simulink model "HevMmReferenceApplication"  (R2020a)
settings: Solver=ode23tb  StartTime=0  StopTime=2474  RelTol=1e-3  EnableMultiTasking=on
undefined symbols (not defined in the file): sigbuilder_block
libraries: autolibshared x2
(part 1 of 2)
settings Model: ModifiedByFormat=The MathWorks, Inc.  SimulationMode=accelerator  PauseTimes=23.46  Creator=The MathWorks, Inc.  LastModifiedBy=The MathWorks, Inc.
settings SolverCC: ZeroCrossAlgorithm=Adaptive  MinimalZcImpactIntegration=on
settings DataIOCC: DSMLogging=off  ReturnWorkspaceOutputs=off
settings DebuggingCC: UnderspecifiedInitializationDetection=Classic  MergeDetectMultiDrivingBlocksExec=none  MaskedZcDiagnostic=none  IgnoredZcDiagnostic=none  ModelReferenceExtraNoncontSigs=none  PregeneratedLibrarySubsystemCodeDiagnostic=none  ArithmeticOperatorsInVariantConditions=warning
settings ModelReferenceCC: UpdateModelReferenceTargets=IfOutOfDate  ModelReferenceMinAlgLoopOccurrences=on  PropagateSignalLabelsOutOfModel=off
settings SFSimCC: SimUseLocalCustomCode=off
settings RTWCC: RTWUseLocalCustomCode=off
settings CodeAppCC: StateflowObjectComments=on
settings GRTTargetCC: TargetLangStandard=C89/C90 (ANSI)
settings ConfigComp: CovMetricSettings=dsw  CovHtmlReporting=on  CovSaveCumulativeToWorkspaceVar=on  CovSaveSingleToWorkspaceVar=on  CovShowResultsExplorer=off  CovExternalEMLEnable=off

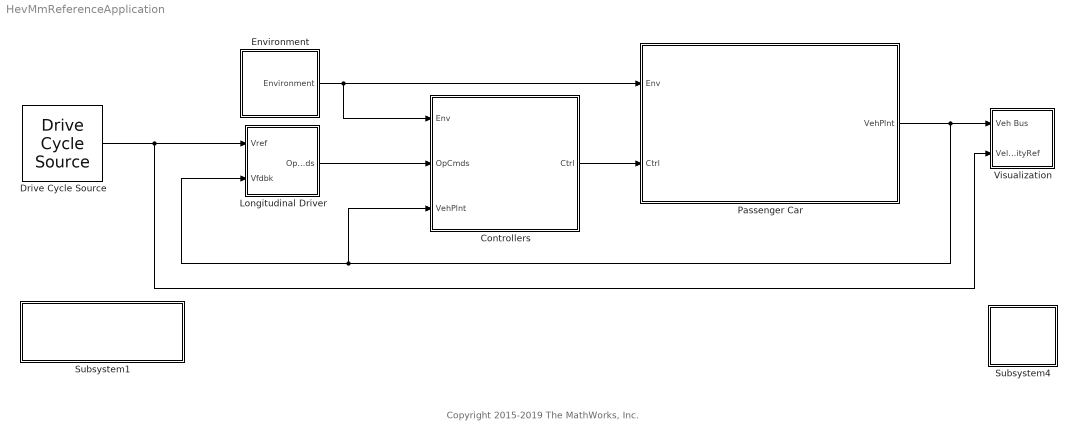
== system HevMmReferenceApplication ==
  note: Copyright 2015-2019 The MathWorks, Inc.
  Controllers : Subsystem
      mask Display: image('SystemControllers.png', 'center')
  Drive Cycle Source : autolibshared/Drive Cycle Source  cycleVar=FTP75  fileVar=L:\Bauto\matlab\test\toolbox\shared\autoblks\scenario\adac.txt  tfinal="2474  seconds"  cycleRepeat=off  outAccPort=off  outGearPort=off  gearList=No gear data  t_wot1=5  xdot_woto=0  xdot_wot1=30  t_wot2=20  xdot_wot2=0  t_wotend=30  srcUnit=m/s  outUnit=m/s  srcAccUnit=m/s/s  outAccUnit=m/s^2  dt=0  aMode=1  faultOption=off  velBnd=2  velBndUnit=mph  inUnit=m/s  timeBnd=1  failOption=off  stopSim=off  maxFaultCnt=10  maxFaultTime=2  maxTotFaultTime=15  traceOption=off  dtTrace=1  traceWindow=10  lastDCname=FTP75 Velocity  lastOutUnit=mph  lastDT=0  lastTB=1  lastSB=2  forceCalcBound=off
      settings: SourceProductBaseCode=PW,MT,VE,VP
  Environment : Subsystem
      mask Display: disp('Environment')
  Longitudinal Driver : Subsystem  Variant=on  VariantControlMode=Label  VariantControl=Variant1  LabelModeActiveChoice=0
      mask Display:
      | if strcmp('1',get_param(gcb,'ActiveVariant'))
      |     disp('Open Loop')
      | else
      |     image('LongitudinalDriver.png','center');
      | end
  Passenger Car : Subsystem
      mask Display: image('PassengerVehicle.png', 'center')
  Subsystem1 : Subsystem
      settings: OpenFcn=edit GenerateEnergyReport
      mask Display: disp('Analyze Power and Energy')
  Subsystem4 : Subsystem
      settings: OpenFcn=helpview([docroot,'/toolbox/autoblks/helptargets.map'], 'hybrid_refapp')
      mask Display: disp('Help')
  Visualization : Subsystem
      mask Display: disp('Visualization')
  wires:
  Longitudinal Driver/1(" OpCmds") -> Controllers/2(OpCmds)
  Drive Cycle Source/1 -> Longitudinal Driver/1("Vref "), Visualization/2(VelocityRef)
  Environment/1(Environment) -> Passenger Car/1(Env), Controllers/1(Env)
  Controllers/1(Ctrl) -> Passenger Car/2(Ctrl)
  Passenger Car/1(VehPlnt) -> Longitudinal Driver/2("Vfdbk "), Controllers/3(VehPlnt), Visualization/1(Veh Bus)

== system HevMmReferenceApplication/Controllers ==
  Env : Inport
  OpCmds : Inport  Port=2
  VehPlnt : Inport  Port=3
  Bus Creator : BusCreator  Inputs=2
  PCM Input : Subsystem
  PCM Output : Subsystem
  Powertrain Control Module (PCM) : Subsystem
  Ctrl : Outport  VectorParamsAs1DForOutWhenUnconnected=off
  wires:
  PCM Output/1(EngCtrl) -> [EngCtrl]
  Bus Creator/1 -> Ctrl/1
  [EngCtrl] -> Bus Creator/1
  [PtCtrl] -> Bus Creator/2
  Env/1 -> [Environment]
  [OpCmds] -> PCM Input/4(OpCmds)
  VehPlnt/1 -> [VehPlnt]
  OpCmds/1 -> [OpCmds]
  [PtCtrl] -> PCM Input/1(PtCtrl)
  [Environment] -> PCM Input/2(Env)
  [VehPlnt] -> PCM Input/3(VehPlnt)
  PCM Output/2(PtCtrl) -> [PtCtrl]
  PCM Input/1(TrqCmd) -> Powertrain Control Module (PCM)/1(TrqCmd)
  PCM Input/2(EngSpd) -> Powertrain Control Module (PCM)/2(EngSpd)
  PCM Input/3(Map) -> Powertrain Control Module (PCM)/3(Map)
  PCM Input/4(Mat) -> Powertrain Control Module (PCM)/4(Mat)
  PCM Input/5(ThrPosPct) -> Powertrain Control Module (PCM)/5(ThrPosPct)
  PCM Input/6(WgAreaPct) -> Powertrain Control Module (PCM)/6(WgAreaPct)
  PCM Input/7(IntkCamPhase) -> Powertrain Control Module (PCM)/7(IntkCamPhase)
  PCM Input/8(ExhCamPhase) -> Powertrain Control Module (PCM)/8(ExhCamPhase)
  PCM Input/9(TurboRackPos) -> Powertrain Control Module (PCM)/9(TurboRackPos)
  PCM Input/10(EgrVlvAreaPct) -> Powertrain Control Module (PCM)/10(EgrVlvAreaPct)
  PCM Input/11(VarCompRatioPos) -> Powertrain Control Module (PCM)/11(VarCompRatioPos)
  PCM Input/12(IntkVlvLift) -> Powertrain Control Module (PCM)/12(IntkVlvLift)
  PCM Input/13(VarIntkRunLen) -> Powertrain Control Module (PCM)/13(VarIntkRunLen)
  PCM Input/14(Afr) -> Powertrain Control Module (PCM)/14(Afr)
  PCM Input/15(IntkSwirlVlvPos) -> Powertrain Control Module (PCM)/15(IntkSwirlVlvPos)
  PCM Input/16(TurboSpd) -> Powertrain Control Module (PCM)/16(TurboSpd)
  PCM Input/17(AmbPrs) -> Powertrain Control Module (PCM)/17(AmbPrs)
  PCM Input/18(AccCmd) -> Powertrain Control Module (PCM)/18(AccCmd)
  PCM Input/19(DecCmd) -> Powertrain Control Module (PCM)/19(DecCmd)
  PCM Input/25(VehSpdFdbk) -> Powertrain Control Module (PCM)/25(VehSpdFdbk)
  PCM Input/26(EngSpdFdbk) -> Powertrain Control Module (PCM)/26(EngSpdFdbk)
  PCM Input/27(EngCltchState) -> Powertrain Control Module (PCM)/27(EngCltchState)
  PCM Input/28(BattSoc) -> Powertrain Control Module (PCM)/28(BattSoc)
  PCM Input/29(BattPwr) -> Powertrain Control Module (PCM)/29(BattPwr)
  PCM Input/30(BattCrnt) -> Powertrain Control Module (PCM)/30(BattCrnt)
  PCM Input/31(EngCltchOutSpd) -> Powertrain Control Module (PCM)/31(EngCltchOutSpd)
  PCM Input/32(MotSpd) -> Powertrain Control Module (PCM)/32(MotSpd)
  PCM Input/33(GenPwrElec) -> Powertrain Control Module (PCM)/33(GenPwrElec)
  PCM Input/34(GenPwrMech) -> Powertrain Control Module (PCM)/34(GenPwrMech)
  PCM Input/20(IgSw) -> Powertrain Control Module (PCM)/20(IgSw)
  PCM Input/22(Ect) -> Powertrain Control Module (PCM)/22(Ect)
  PCM Input/23(EgrDeltaPrs) -> Powertrain Control Module (PCM)/23(EgrVlvDeltaPrs)
  PCM Input/24(EgrInTemp) -> Powertrain Control Module (PCM)/24(EgrVlvInTemp)
  PCM Input/21(Iat) -> Powertrain Control Module (PCM)/21(Iat)
  Powertrain Control Module (PCM)/1(ThrPosPctCmd) -> PCM Output/1(ThrPosPctCmd)
  Powertrain Control Module (PCM)/2(WgAreaPctCmd) -> PCM Output/2(WgAreaPctCmd)
  Powertrain Control Module (PCM)/3(InjPw) -> PCM Output/3(InjPw)
  Powertrain Control Module (PCM)/4(FuelMainSoi) -> PCM Output/4(FuelMainSoi)
  Powertrain Control Module (PCM)/5(SpdAdv) -> PCM Output/5(SpkAdv)
  Powertrain Control Module (PCM)/6(IntkCamPhaseCmd) -> PCM Output/6(IntkCamPhaseCmd)
  Powertrain Control Module (PCM)/7(ExhCamPhaseCmd) -> PCM Output/7(ExhCamPhaseCmd)
  Powertrain Control Module (PCM)/8(TurboRackPosCmd) -> PCM Output/8(TurboRackPosCmd)
  Powertrain Control Module (PCM)/9(EgrVlvAreaPctCmd) -> PCM Output/9(EgrVlvAreaPctCmd)
  Powertrain Control Module (PCM)/10(VarCompRatioPosCmd) -> PCM Output/10(VarCompRatioPosCmd)
  Powertrain Control Module (PCM)/11(IntkVlvLiftCmd) -> PCM Output/11(IntkVlvLiftCmd)
  Powertrain Control Module (PCM)/12(VarIntkRunLenCmd) -> PCM Output/12(VarIntkRunLenCmd)
  Powertrain Control Module (PCM)/13(ClsdLpFuelMult) -> PCM Output/13(ClsdLpFuelMult)
  Powertrain Control Module (PCM)/14(IntkSwirlVlvPosCmd) -> PCM Output/14(IntkSwirlVlvPosCmd)
  Powertrain Control Module (PCM)/15(TrqCmdISC) -> PCM Output/15(TrqCmdISC)
  Powertrain Control Module (PCM)/16(LoadCmd) -> PCM Output/16(LoadCmd)
  Powertrain Control Module (PCM)/17(EstIntkPortFlw) -> PCM Output/17(EstIntkPortFlw)
  Powertrain Control Module (PCM)/18(EngCltchCmd) -> PCM Output/18(EngCltchCmd)
  Powertrain Control Module (PCM)/19(EngTrqCmd) -> PCM Output/19(EngineTrqCmd)
  Powertrain Control Module (PCM)/20(GenTrqCmd) -> PCM Output/20(GenTrqCmd)
  Powertrain Control Module (PCM)/21(MotTrqCmd) -> PCM Output/21(MotTrqCmd)
  Powertrain Control Module (PCM)/22(BrakeCmd) -> PCM Output/22(BrakeCmd)

== system HevMmReferenceApplication/Environment ==
  Bus Creator : BusCreator  Inputs=4
  Bus Creator3 : BusCreator  Inputs=3
  Bus Creator4 : BusCreator  Inputs=2
  Bus Creator5 : BusCreator  Inputs=2
  Constant2 : Constant  Value=0
  Constant3 : Constant  Value=0
  Constant6 : Constant  Value=300
  Constant7 : Constant  Value=101325
  Ground{,1..3} (4 alike) : Ground
  Environment : Outport  VectorParamsAs1DForOutWhenUnconnected=off
  wires:
  Ground2/1 -> Bus Creator5/1  "lam_mu_x"
  Ground3/1 -> Bus Creator5/2  "lam_mu_y"
  Bus Creator5/1 -> Bus Creator4/2  "Ground_mu"
  Bus Creator4/1 -> Bus Creator/3  "Ground"
  Bus Creator3/1 -> Bus Creator/4  "Wind"
  Constant3/1 -> Bus Creator3/1  "wind_x"
  Ground/1 -> Bus Creator3/2  "wind_y"
  Ground1/1 -> Bus Creator3/3  "wind_z"
  Constant6/1 -> Bus Creator/1  "Temp"
  Constant2/1 -> Bus Creator4/1  "Grade"
  Bus Creator/1 -> Environment/1  "Environment"
  Constant7/1 -> Bus Creator/2  "Baro"

== system HevMmReferenceApplication/Longitudinal Driver ==
  note: To switch variants, right-click on this subsystem (from one level above) and chose:
      | Variant, Active choice, <your selection>
  "Vref " : Inport
  "Vfdbk " : Inport  Port=2
  Longitudinal Driver : Subsystem  VariantControl=0
      mask Display: image('LongitudinalDriver.png', 'center')
  Open Loop : Subsystem  VariantControl=1
      mask Display: disp('Open Loop')
  " OpCmds" : Outport  VectorParamsAs1DForOutWhenUnconnected=off

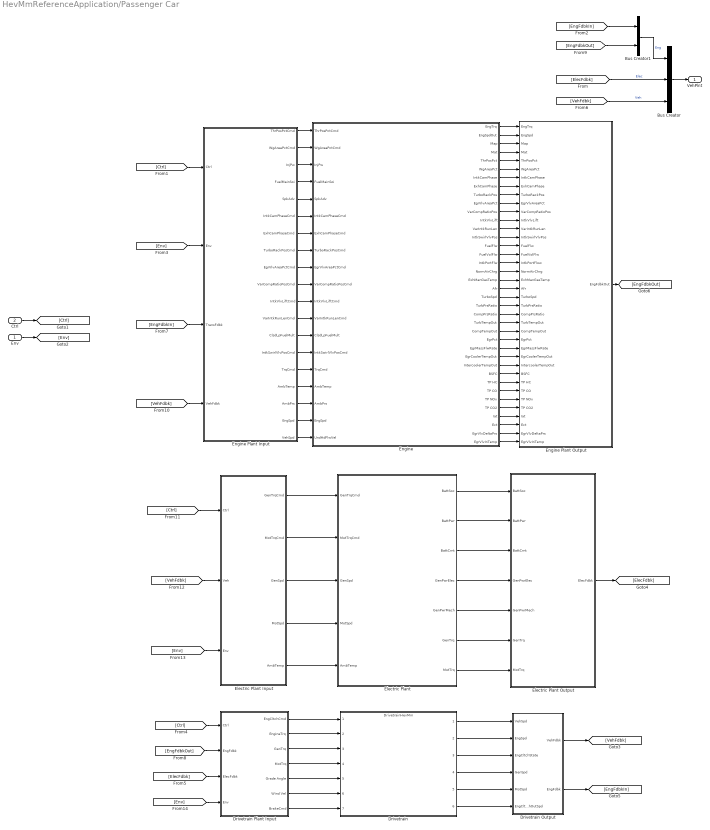
== system HevMmReferenceApplication/Passenger Car ==
  Env : Inport
  Ctrl : Inport  Port=2
  Bus Creator : BusCreator  Inputs=3
  Bus Creator1 : BusCreator  Inputs=2
  Drivetrain : ModelReference  ModelNameDialog=DrivetrainHevMm.slx  SimulationMode=Normal  ModelReferenceVersion=1.434
  Drivetrain Output : Subsystem
  Drivetrain Plant Input : Subsystem
  Electric Plant : Subsystem
  Electric Plant Input : Subsystem
  Electric Plant Output : Subsystem
  Engine : Subsystem  Variant=on  VariantControlMode=Label  LabelModeActiveChoice=SiMappedEngine
  Engine Plant Input : Subsystem
  Engine Plant Output : Subsystem
  VehPlnt : Outport  VectorParamsAs1DForOutWhenUnconnected=off
  wires:
  Ctrl/1 -> [Ctrl]
  Env/1 -> [Env]
  [Ctrl] -> Drivetrain Plant Input/1(Ctrl)
  [EngFdbkOut] -> Drivetrain Plant Input/2(EngFdbk)
  Engine Plant Output/1(EngFdbkOut) -> [EngFdbkOut]
  [Ctrl] -> Engine Plant Input/1(Ctrl)
  [Env] -> Engine Plant Input/2(Env)
  [EngFdbkIn] -> Engine Plant Input/3(TransFdbk)
  [VehFdbk] -> Engine Plant Input/4(VehFdbk)
  Bus Creator/1 -> VehPlnt/1
  [EngFdbkIn] -> Bus Creator1/1
  [VehFdbk] -> Bus Creator/3  "Veh"
  Bus Creator1/1 -> Bus Creator/1  "Eng"
  [EngFdbkOut] -> Bus Creator1/2
  Drivetrain Output/1(VehFdbk) -> [VehFdbk]
  Drivetrain Output/2(EngFdbk) -> [EngFdbkIn]
  Drivetrain/1 -> Drivetrain Output/1(VehSpd)
  Drivetrain/2 -> Drivetrain Output/2("EngSpd ")
  Drivetrain/3 -> Drivetrain Output/3(EngCltchState)
  Drivetrain/4 -> Drivetrain Output/4(GenSpd)
  Electric Plant Output/1(ElecFdbk) -> [ElecFdbk]
  [ElecFdbk] -> Bus Creator/2  "Elec"
  [Ctrl] -> Electric Plant Input/1(Ctrl)
  [ElecFdbk] -> Drivetrain Plant Input/3(ElecFdbk)
  Drivetrain Plant Input/4(MotTrq) -> Drivetrain/4
  Drivetrain Plant Input/3(GenTrq) -> Drivetrain/3
  Drivetrain Plant Input/1(EngCltchCmd) -> Drivetrain/1
  Drivetrain Plant Input/2(EngineTrq) -> Drivetrain/2
  Drivetrain Plant Input/7(BrakeCmd) -> Drivetrain/7
  Drivetrain/5 -> Drivetrain Output/5(MotSpd)
  [VehFdbk] -> Electric Plant Input/2(Veh)
  Drivetrain/6 -> Drivetrain Output/6(EngCltchOutSpd)
  Electric Plant Input/1(GenTrqCmd) -> Electric Plant/1(GenTrqCmd)
  Electric Plant Input/2(MotTrqCmd) -> Electric Plant/2(MotTrqCmd)
  Electric Plant Input/3(GenSpd) -> Electric Plant/3(GenSpd)
  Electric Plant Input/4(MotSpd) -> Electric Plant/4(MotSpd)
  Electric Plant/1(BattSoc) -> Electric Plant Output/1(BattSoc)
  Electric Plant/2(BattPwr) -> Electric Plant Output/2(BattPwr)
  Electric Plant/3(BattCrnt) -> Electric Plant Output/3(BattCrnt)
  Electric Plant/4(GenPwrElec) -> Electric Plant Output/4(GenPwrElec)
  Electric Plant/5(GenPwrMech) -> Electric Plant Output/5(GenPwrMech)
  Electric Plant/6(GenTrq) -> Electric Plant Output/6(GenTrq)
  Electric Plant/7(MotTrq) -> Electric Plant Output/7(MotTrq)
  [Env] -> Electric Plant Input/3(Env)
  Electric Plant Input/5(AmbTemp) -> Electric Plant/5(AmbTemp)
  [Env] -> Drivetrain Plant Input/4(Env)
  Drivetrain Plant Input/5(Grade Angle) -> Drivetrain/5
  Drivetrain Plant Input/6(Wind Vel) -> Drivetrain/6
  Engine Plant Input/19(VehSpd) -> Engine/19(UndHdFlwVel)
  Engine Plant Input/16(AmbTemp) -> Engine/16(AmbTemp)
  Engine Plant Input/13(ClsdLpFuelMult) -> Engine/13(ClsdLpFuelMult)
  Engine Plant Input/12(VarIntkRunLenCmd) -> Engine/12(VarIntkRunLenCmd)
  Engine Plant Input/14(IntkSwirlVlvPosCmd) -> Engine/14(IntkSwirlVlvPosCmd)
  Engine Plant Input/9(EgrVlvAreaPctCmd) -> Engine/9(EgrVlvAreaPctCmd)
  Engine Plant Input/5(SpkAdv) -> Engine/5(SpkAdv)
  Engine Plant Input/4(FuelMainSoi) -> Engine/4(FuelMainSoi)
  Engine Plant Input/18(EngSpd) -> Engine/18(EngSpd)
  Engine Plant Input/10(VarCompRatioPosCmd) -> Engine/10(VarCompRatioPosCmd)
  Engine Plant Input/7(ExhCamPhaseCmd) -> Engine/7(ExhCamPhaseCmd)
  Engine Plant Input/6(IntkCamPhaseCmd) -> Engine/6(IntkCamPhaseCmd)
  Engine Plant Input/2(WgAreaPctCmd) -> Engine/2(WgAreaPctCmd)
  Engine Plant Input/8(TurboRackPosCmd) -> Engine/8(TurboRackPosCmd)
  Engine Plant Input/15(TrqCmd) -> Engine/15(TrqCmd)
  Engine Plant Input/3(InjPw) -> Engine/3(InjPw)
  Engine Plant Input/17(AmbPrs) -> Engine/17(AmbPrs)
  Engine Plant Input/11(IntkVlvLiftCmd) -> Engine/11(IntkVlvLiftCmd)
  Engine Plant Input/1(ThrPosPctCmd) -> Engine/1(ThrPosPctCmd)
  Engine/17(IntkPortFlw) -> Engine Plant Output/17(IntkPortFlow)
  Engine/16(FuelVolFlw) -> Engine Plant Output/16(FuelVolFlw)
  Engine/18(NormAirChrg) -> Engine Plant Output/18(NormAirChrg)
  Engine/15(FuelFlw) -> Engine Plant Output/15(FuelFlw)
  Engine/19(ExhManGasTemp) -> Engine Plant Output/19(ExhManGasTemp)
  Engine/14(IntkSwirlVlvPos) -> Engine Plant Output/14(IntkSwirlVlvPos)
  Engine/20(Afr) -> Engine Plant Output/20(Afr)
  Engine/21(TurboSpd) -> Engine Plant Output/21(TurboSpd)
  Engine/13(VarIntkRunLen) -> Engine Plant Output/13(VarIntkRunLen)
  Engine/22(TurbPrsRatio) -> Engine Plant Output/22(TurbPrsRatio)
  Engine/12(IntkVlvLift) -> Engine Plant Output/12(IntkVlvLift)
  Engine/23(CompPrsRatio) -> Engine Plant Output/23(CompPrsRatio)
  Engine/11(VarCompRatioPos) -> Engine Plant Output/11(VarCompRatioPos)
  Engine/24(TurbTempOut) -> Engine Plant Output/24(TurbTempOut)
  Engine/10(EgrVlvAreaPct) -> Engine Plant Output/10(EgrVlvAreaPct)
  Engine/25(CompTempOut) -> Engine Plant Output/25(CompTempOut)
  Engine/9(TurboRackPos) -> Engine Plant Output/9(TurboRackPos)
  Engine/26(EgrPct) -> Engine Plant Output/26(EgrPct)
  Engine/8(ExhCamPhase) -> Engine Plant Output/8(ExhCamPhase)
  Engine/27(EgrMassFlwRate) -> Engine Plant Output/27(EgrMassFlwRate)
  Engine/7(IntkCamPhase) -> Engine Plant Output/7(IntkCamPhase)
  Engine/28(EgrCoolerTempOut) -> Engine Plant Output/28(EgrCoolerTempOut)
  Engine/6(WgAreaPct) -> Engine Plant Output/6(WgAreaPct)
  Engine/29(IntercoolerTempOut) -> Engine Plant Output/29(IntercoolerTempOut)
  Engine/5(ThrPosPct) -> Engine Plant Output/5(ThrPosPct)
  Engine/30(BSFC) -> Engine Plant Output/30(BSFC)
  Engine/4(Mat) -> Engine Plant Output/4(Mat)
  Engine/31(TP HC) -> Engine Plant Output/31(TP HC)
  Engine/3(Map) -> Engine Plant Output/3(Map)
  Engine/32(TP CO) -> Engine Plant Output/32(TP CO)
  Engine/2(EngSpdOut) -> Engine Plant Output/2(EngSpd)
  Engine/33(TP NOx) -> Engine Plant Output/33(TP NOx)
  Engine/1(EngTrq) -> Engine Plant Output/1(EngTrq)
  Engine/34(TP CO2) -> Engine Plant Output/34(TP CO2)
  Engine/35(Iat) -> Engine Plant Output/35(Iat)
  Engine/36(Ect) -> Engine Plant Output/36(Ect)
  Engine/37(EgrVlvDeltaPrs) -> Engine Plant Output/37(EgrVlvDeltaPrs)
  Engine/38(EgrVlvInTemp) -> Engine Plant Output/38(EgrVlvInTemp)

== system HevMmReferenceApplication/Subsystem1 ==

== system HevMmReferenceApplication/Subsystem4 ==

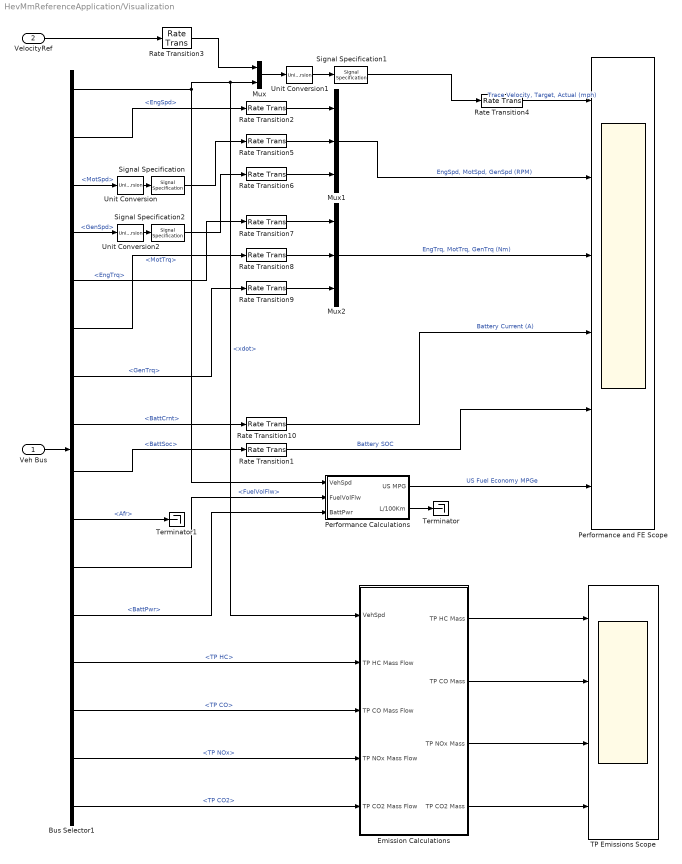
== system HevMmReferenceApplication/Visualization ==
  Veh Bus : Inport
  VelocityRef : Inport  Port=2
  Bus Selector1 : BusSelector  OutputSignals=Veh.xdot,Eng.EngFdbkOut.EngSpd,Veh.MotSpd,Veh.GenSpd,Eng.EngFdbkOut.EngTrq,Elec.MotTrq,Elec.GenTrq,Elec.BattCrnt,Elec.BattSoc,Eng.EngFdbkOut.Afr,Eng.EngFdbkOut.FuelVolFlw,Elec.BattPwr,Eng.EngFdbkOut.TP HC,Eng.EngFdbkOut.TP CO,Eng.EngFdbkOut.TP NOx,Eng.EngFdbkOut.TP CO2
  Emission Calculations : Subsystem
  Mux : Mux  Inputs=2
  Mux1 : Mux  Inputs=3
  Mux2 : Mux  Inputs=3
  Performance Calculations : Subsystem
  Performance and FE Scope : Scope  NumInputPorts=6
  Rate Transition{1..10} (10 alike) : RateTransition  Deterministic=off
  Signal Specification : SignalSpecification  Unit=rpm
  Signal Specification1 : SignalSpecification  Unit=mph
  Signal Specification2 : SignalSpecification  Unit=rpm
  TP Emissions Scope : Scope  NumInputPorts=4
  Terminator : Terminator
  Terminator1 : Terminator
  Unit Conversion : UnitConversion
  Unit Conversion1 : UnitConversion
  Unit Conversion2 : UnitConversion
  wires:
  Veh Bus/1 -> Bus Selector1/1
  Bus Selector1/1 -> Mux/2, Emission Calculations/1(VehSpd), Performance Calculations/1(VehSpd)  "<xdot>"
  Bus Selector1/2 -> Rate Transition2/1  "<EngSpd>"
  Mux/1 -> Unit Conversion1/1
  Bus Selector1/11 -> Performance Calculations/2(FuelVolFlw)  "<FuelVolFlw>"
  Performance Calculations/1(US MPG) -> Performance and FE Scope/6  "US Fuel Economy MPGe"
  Performance Calculations/2(L/100Km) -> Terminator/1
  Bus Selector1/10 -> Terminator1/1  "<Afr>"
  Signal Specification1/1 -> Rate Transition4/1
  VelocityRef/1 -> Rate Transition3/1
  Bus Selector1/9 -> Rate Transition1/1  "<BattSoc>"
  Bus Selector1/13 -> Emission Calculations/2(TP HC Mass Flow)  "<TP HC>"
  Bus Selector1/14 -> Emission Calculations/3(TP CO Mass Flow)  "<TP CO>"
  Bus Selector1/15 -> Emission Calculations/4(TP NOx Mass Flow)  "<TP NOx>"
  Emission Calculations/1(TP HC Mass) -> TP Emissions Scope/1
  Emission Calculations/2(TP CO Mass) -> TP Emissions Scope/2
  Emission Calculations/3(TP NOx Mass) -> TP Emissions Scope/3
  Bus Selector1/16 -> Emission Calculations/5(TP CO2 Mass Flow)  "<TP CO2>"
  Emission Calculations/4(TP CO2 Mass) -> TP Emissions Scope/4
  Rate Transition3/1 -> Mux/1
  Rate Transition1/1 -> Performance and FE Scope/5  "Battery SOC"
  Mux1/1 -> Performance and FE Scope/2  "EngSpd, MotSpd, GenSpd (RPM)"
  Rate Transition4/1 -> Performance and FE Scope/1  "Trace Velocity, Target, Actual (mph)"
  Bus Selector1/12 -> Performance Calculations/3(BattPwr)  "<BattPwr>"
  Bus Selector1/3 -> Unit Conversion/1  "<MotSpd>"
  Bus Selector1/4 -> Unit Conversion2/1  "<GenSpd>"
  Rate Transition2/1 -> Mux1/1
  Rate Transition5/1 -> Mux1/2
  Rate Transition6/1 -> Mux1/3
  Rate Transition9/1 -> Mux2/3
  Rate Transition8/1 -> Mux2/2
  Rate Transition7/1 -> Mux2/1
  Mux2/1 -> Performance and FE Scope/3  "EngTrq, MotTrq, GenTrq (Nm)"
  Bus Selector1/5 -> Rate Transition7/1  "<EngTrq>"
  Bus Selector1/6 -> Rate Transition8/1  "<MotTrq>"
  Bus Selector1/7 -> Rate Transition9/1  "<GenTrq>"
  Bus Selector1/8 -> Rate Transition10/1  "<BattCrnt>"
  Rate Transition10/1 -> Performance and FE Scope/4  "Battery Current (A)"
  Signal Specification/1 -> Rate Transition5/1
  Signal Specification2/1 -> Rate Transition6/1
  Unit Conversion/1 -> Signal Specification/1
  Unit Conversion1/1 -> Signal Specification1/1
  Unit Conversion2/1 -> Signal Specification2/1

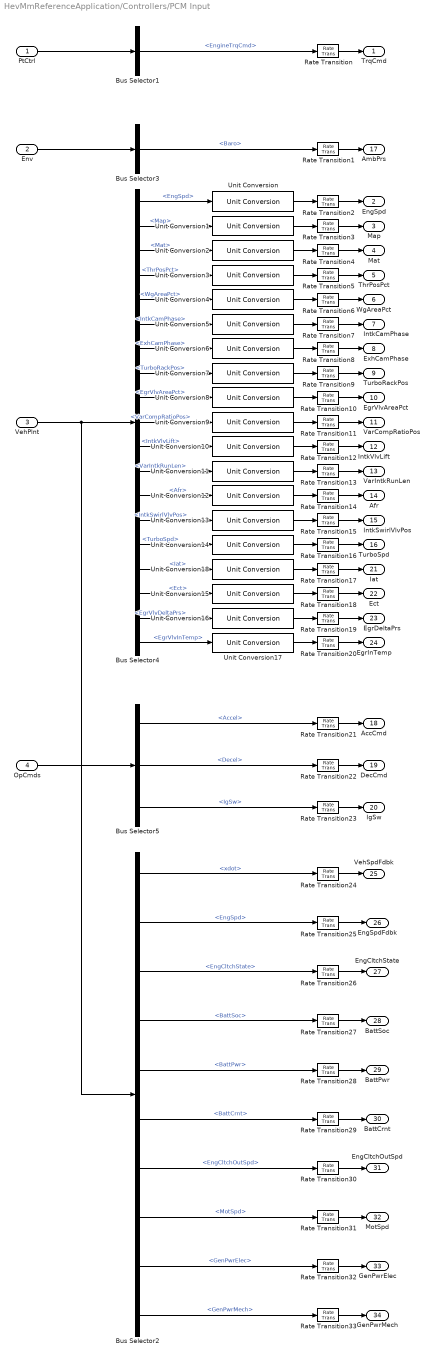
== system HevMmReferenceApplication/Controllers/PCM Input ==
  PtCtrl : Inport
  Env : Inport  Port=2
  VehPlnt : Inport  Port=3
  OpCmds : Inport  Port=4
  Bus Selector1 : BusSelector  OutputSignals=EngineTrqCmd
  Bus Selector2 : BusSelector  OutputSignals=Veh.xdot,Eng.EngFdbk.EngSpd,Veh.EngCltchState,Elec.BattSoc,Elec.BattPwr,Elec.BattCrnt,Veh.EngCltchOutSpd,Veh.MotSpd,Elec.GenPwrElec,Elec.GenPwrMech
  Bus Selector3 : BusSelector  OutputSignals=Baro
  Bus Selector4 : BusSelector  OutputSignals=Eng.EngFdbkOut.EngSpd,Eng.EngFdbkOut.Map,Eng.EngFdbkOut.Mat,Eng.EngFdbkOut.ThrPosPct,Eng.EngFdbkOut.WgAreaPct,Eng.EngFdbkOut.IntkCamPhase,Eng.EngFdbkOut.ExhCamPhase,Eng.EngFdbkOut.TurboRackPos,Eng.EngFdbkOut.EgrVlvAreaPct,Eng.EngFdbkOut.VarCompRatioPos,Eng.EngFdbkOut.IntkVlvLift,Eng.EngFdbkOut.VarIntkRunLen,Eng.EngFdbkOut.Afr,Eng.EngFdbkOut.IntkSwirlVlvPos,Eng.EngFdbkOut.TurboSpd,Eng.EngFdbkOut.Iat,Eng.EngFdbkOut.Ect,Eng.EngFdbkOut.EgrVlvDeltaPrs,Eng.EngFdbkOut.EgrVlvInTemp
  Bus Selector5 : BusSelector  OutputSignals=Info.Accel,Info.Decel,IgSw
  Rate Transition{,1..33} (34 alike) : RateTransition
  Unit Conversion{,1..18} (19 alike) : UnitConversion
  TrqCmd : Outport  VectorParamsAs1DForOutWhenUnconnected=off
  EngSpd : Outport  Port=2  VectorParamsAs1DForOutWhenUnconnected=off
  Map : Outport  Port=3  VectorParamsAs1DForOutWhenUnconnected=off
  Mat : Outport  Port=4  VectorParamsAs1DForOutWhenUnconnected=off
  ThrPosPct : Outport  Port=5  VectorParamsAs1DForOutWhenUnconnected=off
  WgAreaPct : Outport  Port=6  VectorParamsAs1DForOutWhenUnconnected=off
  IntkCamPhase : Outport  Port=7  VectorParamsAs1DForOutWhenUnconnected=off
  ExhCamPhase : Outport  Port=8  VectorParamsAs1DForOutWhenUnconnected=off
  TurboRackPos : Outport  Port=9  VectorParamsAs1DForOutWhenUnconnected=off
  EgrVlvAreaPct : Outport  Port=10  VectorParamsAs1DForOutWhenUnconnected=off
  VarCompRatioPos : Outport  Port=11  VectorParamsAs1DForOutWhenUnconnected=off
  IntkVlvLift : Outport  Port=12  VectorParamsAs1DForOutWhenUnconnected=off
  VarIntkRunLen : Outport  Port=13  VectorParamsAs1DForOutWhenUnconnected=off
  Afr : Outport  Port=14  VectorParamsAs1DForOutWhenUnconnected=off
  IntkSwirlVlvPos : Outport  Port=15  VectorParamsAs1DForOutWhenUnconnected=off
  TurboSpd : Outport  Port=16  VectorParamsAs1DForOutWhenUnconnected=off
  AmbPrs : Outport  Port=17  VectorParamsAs1DForOutWhenUnconnected=off
  AccCmd : Outport  Port=18  VectorParamsAs1DForOutWhenUnconnected=off
  DecCmd : Outport  Port=19  VectorParamsAs1DForOutWhenUnconnected=off
  IgSw : Outport  Port=20  VectorParamsAs1DForOutWhenUnconnected=off
  Iat : Outport  Port=21  VectorParamsAs1DForOutWhenUnconnected=off
  Ect : Outport  Port=22  VectorParamsAs1DForOutWhenUnconnected=off
  EgrDeltaPrs : Outport  Port=23  VectorParamsAs1DForOutWhenUnconnected=off
  EgrInTemp : Outport  Port=24  VectorParamsAs1DForOutWhenUnconnected=off
  VehSpdFdbk : Outport  Port=25  VectorParamsAs1DForOutWhenUnconnected=off
  EngSpdFdbk : Outport  Port=26  VectorParamsAs1DForOutWhenUnconnected=off
  EngCltchState : Outport  Port=27  VectorParamsAs1DForOutWhenUnconnected=off
  BattSoc : Outport  Port=28  VectorParamsAs1DForOutWhenUnconnected=off
  BattPwr : Outport  Port=29  VectorParamsAs1DForOutWhenUnconnected=off
  BattCrnt : Outport  Port=30  VectorParamsAs1DForOutWhenUnconnected=off
  EngCltchOutSpd : Outport  Port=31  VectorParamsAs1DForOutWhenUnconnected=off
  MotSpd : Outport  Port=32  VectorParamsAs1DForOutWhenUnconnected=off
  GenPwrElec : Outport  Port=33  VectorParamsAs1DForOutWhenUnconnected=off
  GenPwrMech : Outport  Port=34  VectorParamsAs1DForOutWhenUnconnected=off
  wires:
  PtCtrl/1 -> Bus Selector1/1
  OpCmds/1 -> Bus Selector5/1
  VehPlnt/1 -> Bus Selector4/1, Bus Selector2/1
  Unit Conversion6/1 -> Rate Transition8/1
  Unit Conversion1/1 -> Rate Transition3/1
  Unit Conversion14/1 -> Rate Transition16/1
  Unit Conversion12/1 -> Rate Transition14/1
  Unit Conversion2/1 -> Rate Transition4/1
  Unit Conversion13/1 -> Rate Transition15/1
  Unit Conversion7/1 -> Rate Transition9/1
  Unit Conversion4/1 -> Rate Transition6/1
  Unit Conversion3/1 -> Rate Transition5/1
  Unit Conversion5/1 -> Rate Transition7/1
  Unit Conversion10/1 -> Rate Transition12/1
  Unit Conversion11/1 -> Rate Transition13/1
  Unit Conversion/1 -> Rate Transition2/1
  Unit Conversion9/1 -> Rate Transition11/1
  Unit Conversion8/1 -> Rate Transition10/1
  Unit Conversion15/1 -> Rate Transition18/1
  Env/1 -> Bus Selector3/1
  Unit Conversion17/1 -> Rate Transition20/1
  Unit Conversion16/1 -> Rate Transition19/1
  Unit Conversion18/1 -> Rate Transition17/1
  Bus Selector3/1 -> Rate Transition1/1  "<Baro>"
  Bus Selector4/1 -> Unit Conversion/1  "<EngSpd>"
  Bus Selector4/2 -> Unit Conversion1/1  "<Map>"
  Bus Selector4/3 -> Unit Conversion2/1  "<Mat>"
  Bus Selector4/4 -> Unit Conversion3/1  "<ThrPosPct>"
  Bus Selector4/5 -> Unit Conversion4/1  "<WgAreaPct>"
  Bus Selector4/6 -> Unit Conversion5/1  "<IntkCamPhase>"
  Bus Selector4/7 -> Unit Conversion6/1  "<ExhCamPhase>"
  Bus Selector4/8 -> Unit Conversion7/1  "<TurboRackPos>"
  Bus Selector4/9 -> Unit Conversion8/1  "<EgrVlvAreaPct>"
  Bus Selector4/10 -> Unit Conversion9/1  "<VarCompRatioPos>"
  Bus Selector4/11 -> Unit Conversion10/1  "<IntkVlvLift>"
  Bus Selector4/12 -> Unit Conversion11/1  "<VarIntkRunLen>"
  Bus Selector4/13 -> Unit Conversion12/1  "<Afr>"
  Bus Selector4/14 -> Unit Conversion13/1  "<IntkSwirlVlvPos>"
  Bus Selector4/15 -> Unit Conversion14/1  "<TurboSpd>"
  Bus Selector4/16 -> Unit Conversion18/1  "<Iat>"
  Bus Selector4/17 -> Unit Conversion15/1  "<Ect>"
  Bus Selector4/18 -> Unit Conversion16/1  "<EgrVlvDeltaPrs>"
  Bus Selector4/19 -> Unit Conversion17/1  "<EgrVlvInTemp>"
  Bus Selector5/1 -> Rate Transition21/1  "<Accel>"
  Bus Selector5/2 -> Rate Transition22/1  "<Decel>"
  Bus Selector5/3 -> Rate Transition23/1  "<IgSw>"
  Bus Selector2/1 -> Rate Transition24/1  "<xdot>"
  Bus Selector2/2 -> Rate Transition25/1  "<EngSpd>"
  Bus Selector2/3 -> Rate Transition26/1  "<EngCltchState>"
  Bus Selector2/4 -> Rate Transition27/1  "<BattSoc>"
  Bus Selector2/5 -> Rate Transition28/1  "<BattPwr>"
  Bus Selector2/6 -> Rate Transition29/1  "<BattCrnt>"
  Bus Selector2/7 -> Rate Transition30/1  "<EngCltchOutSpd>"
  Bus Selector2/8 -> Rate Transition31/1  "<MotSpd>"
  Bus Selector2/9 -> Rate Transition32/1  "<GenPwrElec>"
  Bus Selector2/10 -> Rate Transition33/1  "<GenPwrMech>"
  Bus Selector1/1 -> Rate Transition/1  "<EngineTrqCmd>"
  Rate Transition10/1 -> EgrVlvAreaPct/1
  Rate Transition1/1 -> AmbPrs/1
  Rate Transition12/1 -> IntkVlvLift/1
  Rate Transition11/1 -> VarCompRatioPos/1
  Rate Transition13/1 -> VarIntkRunLen/1
  Rate Transition15/1 -> IntkSwirlVlvPos/1
  Rate Transition14/1 -> Afr/1
  Rate Transition16/1 -> TurboSpd/1
  Rate Transition19/1 -> EgrDeltaPrs/1
  Rate Transition17/1 -> Iat/1
  Rate Transition18/1 -> Ect/1
  Rate Transition2/1 -> EngSpd/1
  Rate Transition3/1 -> Map/1
  Rate Transition20/1 -> EgrInTemp/1
  Rate Transition4/1 -> Mat/1
  Rate Transition5/1 -> ThrPosPct/1
  Rate Transition6/1 -> WgAreaPct/1
  Rate Transition9/1 -> TurboRackPos/1
  Rate Transition7/1 -> IntkCamPhase/1
  Rate Transition8/1 -> ExhCamPhase/1
  Rate Transition/1 -> TrqCmd/1
  Rate Transition21/1 -> AccCmd/1
  Rate Transition22/1 -> DecCmd/1
  Rate Transition23/1 -> IgSw/1
  Rate Transition24/1 -> VehSpdFdbk/1
  Rate Transition25/1 -> EngSpdFdbk/1
  Rate Transition26/1 -> EngCltchState/1
  Rate Transition27/1 -> BattSoc/1
  Rate Transition28/1 -> BattPwr/1
  Rate Transition30/1 -> EngCltchOutSpd/1
  Rate Transition29/1 -> BattCrnt/1
  Rate Transition31/1 -> MotSpd/1
  Rate Transition32/1 -> GenPwrElec/1
  Rate Transition33/1 -> GenPwrMech/1

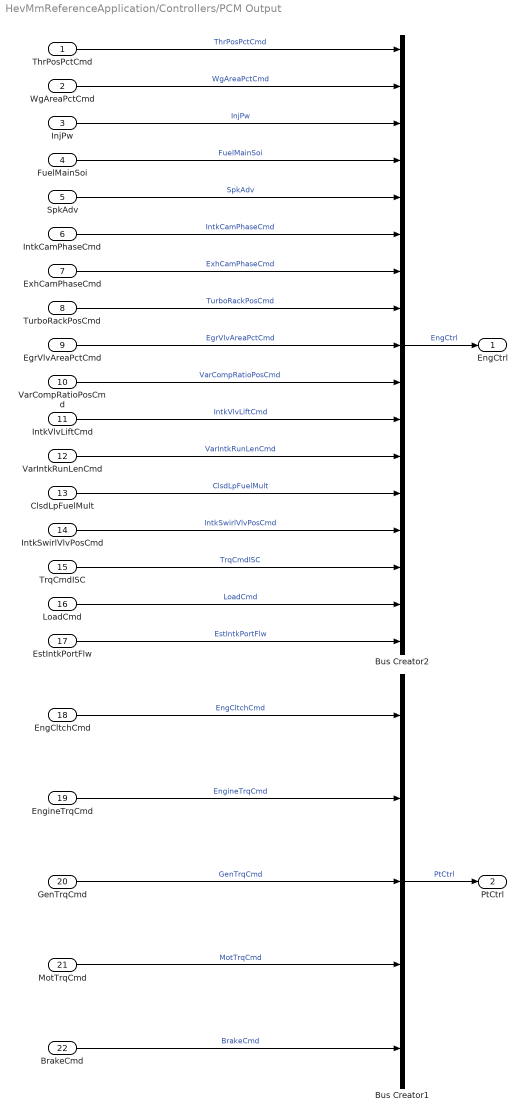
== system HevMmReferenceApplication/Controllers/PCM Output ==
  ThrPosPctCmd : Inport
  WgAreaPctCmd : Inport  Port=2
  InjPw : Inport  Port=3
  FuelMainSoi : Inport  Port=4
  SpkAdv : Inport  Port=5
  IntkCamPhaseCmd : Inport  Port=6
  ExhCamPhaseCmd : Inport  Port=7
  TurboRackPosCmd : Inport  Port=8
  EgrVlvAreaPctCmd : Inport  Port=9
  VarCompRatioPosCmd : Inport  Port=10
  IntkVlvLiftCmd : Inport  Port=11
  VarIntkRunLenCmd : Inport  Port=12
  ClsdLpFuelMult : Inport  Port=13
  IntkSwirlVlvPosCmd : Inport  Port=14
  TrqCmdISC : Inport  Port=15
  LoadCmd : Inport  Port=16
  EstIntkPortFlw : Inport  Port=17
  EngCltchCmd : Inport  Port=18
  EngineTrqCmd : Inport  Port=19
  GenTrqCmd : Inport  Port=20
  MotTrqCmd : Inport  Port=21
  BrakeCmd : Inport  Port=22
  Bus Creator1 : BusCreator  Inputs=5
  Bus Creator2 : BusCreator  Inputs=17
  EngCtrl : Outport  VectorParamsAs1DForOutWhenUnconnected=off
  PtCtrl : Outport  Port=2  VectorParamsAs1DForOutWhenUnconnected=off
  wires:
  BrakeCmd/1 -> Bus Creator1/5  "BrakeCmd"
  Bus Creator1/1 -> PtCtrl/1  "PtCtrl"
  EngCltchCmd/1 -> Bus Creator1/1  "EngCltchCmd"
  EngineTrqCmd/1 -> Bus Creator1/2  "EngineTrqCmd"
  GenTrqCmd/1 -> Bus Creator1/3  "GenTrqCmd"
  MotTrqCmd/1 -> Bus Creator1/4  "MotTrqCmd"
  Bus Creator2/1 -> EngCtrl/1  "EngCtrl"
  LoadCmd/1 -> Bus Creator2/16  "LoadCmd"
  TurboRackPosCmd/1 -> Bus Creator2/8  "TurboRackPosCmd"
  InjPw/1 -> Bus Creator2/3  "InjPw"
  IntkSwirlVlvPosCmd/1 -> Bus Creator2/14  "IntkSwirlVlvPosCmd"
  FuelMainSoi/1 -> Bus Creator2/4  "FuelMainSoi"
  ThrPosPctCmd/1 -> Bus Creator2/1  "ThrPosPctCmd"
  VarIntkRunLenCmd/1 -> Bus Creator2/12  "VarIntkRunLenCmd"
  TrqCmdISC/1 -> Bus Creator2/15  "TrqCmdISC"
  IntkCamPhaseCmd/1 -> Bus Creator2/6  "IntkCamPhaseCmd"
  EgrVlvAreaPctCmd/1 -> Bus Creator2/9  "EgrVlvAreaPctCmd"
  WgAreaPctCmd/1 -> Bus Creator2/2  "WgAreaPctCmd"
  SpkAdv/1 -> Bus Creator2/5  "SpkAdv"
  EstIntkPortFlw/1 -> Bus Creator2/17  "EstIntkPortFlw"
  ClsdLpFuelMult/1 -> Bus Creator2/13  "ClsdLpFuelMult"
  VarCompRatioPosCmd/1 -> Bus Creator2/10  "VarCompRatioPosCmd"
  ExhCamPhaseCmd/1 -> Bus Creator2/7  "ExhCamPhaseCmd"
  IntkVlvLiftCmd/1 -> Bus Creator2/11  "IntkVlvLiftCmd"

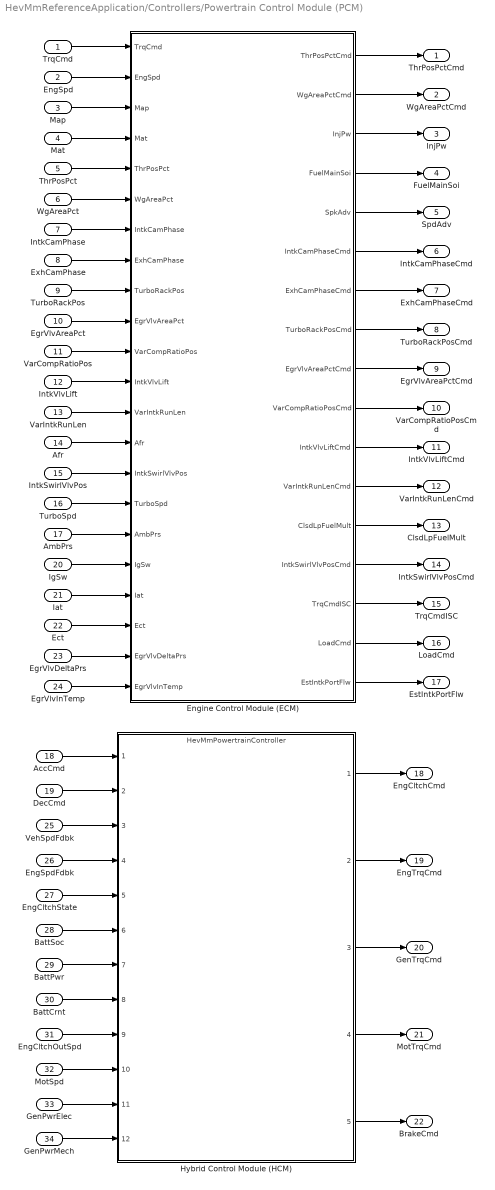
== system HevMmReferenceApplication/Controllers/Powertrain Control Module (PCM) ==
  TrqCmd : Inport
  EngSpd : Inport  Port=2
  Map : Inport  Port=3
  Mat : Inport  Port=4
  ThrPosPct : Inport  Port=5
  WgAreaPct : Inport  Port=6
  IntkCamPhase : Inport  Port=7
  ExhCamPhase : Inport  Port=8
  TurboRackPos : Inport  Port=9
  EgrVlvAreaPct : Inport  Port=10
  VarCompRatioPos : Inport  Port=11
  IntkVlvLift : Inport  Port=12
  VarIntkRunLen : Inport  Port=13
  Afr : Inport  Port=14
  IntkSwirlVlvPos : Inport  Port=15
  TurboSpd : Inport  Port=16
  AmbPrs : Inport  Port=17
  AccCmd : Inport  Port=18
  DecCmd : Inport  Port=19
  IgSw : Inport  Port=20
  Iat : Inport  Port=21
  Ect : Inport  Port=22
  EgrVlvDeltaPrs : Inport  Port=23
  EgrVlvInTemp : Inport  Port=24
  VehSpdFdbk : Inport  Port=25
  EngSpdFdbk : Inport  Port=26
  EngCltchState : Inport  Port=27
  BattSoc : Inport  Port=28
  BattPwr : Inport  Port=29
  BattCrnt : Inport  Port=30
  EngCltchOutSpd : Inport  Port=31
  MotSpd : Inport  Port=32
  GenPwrElec : Inport  Port=33
  GenPwrMech : Inport  Port=34
  Engine Control Module (ECM) : Subsystem  Variant=on  VariantControlMode=Label  LabelModeActiveChoice=SiEngineController
  Hybrid Control Module (HCM) : ModelReference  ModelNameDialog=HevMmPowertrainController.slx  ModelReferenceVersion=1.829
  ThrPosPctCmd : Outport  VectorParamsAs1DForOutWhenUnconnected=off
  WgAreaPctCmd : Outport  Port=2  VectorParamsAs1DForOutWhenUnconnected=off
  InjPw : Outport  Port=3  VectorParamsAs1DForOutWhenUnconnected=off
  FuelMainSoi : Outport  Port=4  VectorParamsAs1DForOutWhenUnconnected=off
  SpdAdv : Outport  Port=5  VectorParamsAs1DForOutWhenUnconnected=off
  IntkCamPhaseCmd : Outport  Port=6  VectorParamsAs1DForOutWhenUnconnected=off
  ExhCamPhaseCmd : Outport  Port=7  VectorParamsAs1DForOutWhenUnconnected=off
  TurboRackPosCmd : Outport  Port=8  VectorParamsAs1DForOutWhenUnconnected=off
  EgrVlvAreaPctCmd : Outport  Port=9  VectorParamsAs1DForOutWhenUnconnected=off
  VarCompRatioPosCmd : Outport  Port=10  VectorParamsAs1DForOutWhenUnconnected=off
  IntkVlvLiftCmd : Outport  Port=11  VectorParamsAs1DForOutWhenUnconnected=off
  VarIntkRunLenCmd : Outport  Port=12  VectorParamsAs1DForOutWhenUnconnected=off
  ClsdLpFuelMult : Outport  Port=13  VectorParamsAs1DForOutWhenUnconnected=off
  IntkSwirlVlvPosCmd : Outport  Port=14  VectorParamsAs1DForOutWhenUnconnected=off
  TrqCmdISC : Outport  Port=15  VectorParamsAs1DForOutWhenUnconnected=off
  LoadCmd : Outport  Port=16  VectorParamsAs1DForOutWhenUnconnected=off
  EstIntkPortFlw : Outport  Port=17  VectorParamsAs1DForOutWhenUnconnected=off
  EngCltchCmd : Outport  Port=18  VectorParamsAs1DForOutWhenUnconnected=off
  EngTrqCmd : Outport  Port=19  VectorParamsAs1DForOutWhenUnconnected=off
  GenTrqCmd : Outport  Port=20  VectorParamsAs1DForOutWhenUnconnected=off
  MotTrqCmd : Outport  Port=21  VectorParamsAs1DForOutWhenUnconnected=off
  BrakeCmd : Outport  Port=22  VectorParamsAs1DForOutWhenUnconnected=off
  wires:
  BattSoc/1 -> Hybrid Control Module (HCM)/6
  GenPwrMech/1 -> Hybrid Control Module (HCM)/12
  VehSpdFdbk/1 -> Hybrid Control Module (HCM)/3
  Hybrid Control Module (HCM)/2 -> EngTrqCmd/1
  Hybrid Control Module (HCM)/5 -> BrakeCmd/1
  Hybrid Control Module (HCM)/3 -> GenTrqCmd/1
  MotSpd/1 -> Hybrid Control Module (HCM)/10
  GenPwrElec/1 -> Hybrid Control Module (HCM)/11
  EngCltchOutSpd/1 -> Hybrid Control Module (HCM)/9
  Hybrid Control Module (HCM)/4 -> MotTrqCmd/1
  Hybrid Control Module (HCM)/1 -> EngCltchCmd/1
  EngCltchState/1 -> Hybrid Control Module (HCM)/5
  BattPwr/1 -> Hybrid Control Module (HCM)/7
  BattCrnt/1 -> Hybrid Control Module (HCM)/8
  AccCmd/1 -> Hybrid Control Module (HCM)/1
  EngSpdFdbk/1 -> Hybrid Control Module (HCM)/4
  DecCmd/1 -> Hybrid Control Module (HCM)/2
  VarCompRatioPos/1 -> Engine Control Module (ECM)/11(VarCompRatioPos)
  IntkVlvLift/1 -> Engine Control Module (ECM)/12(IntkVlvLift)
  VarIntkRunLen/1 -> Engine Control Module (ECM)/13(VarIntkRunLen)
  Afr/1 -> Engine Control Module (ECM)/14(Afr)
  IntkSwirlVlvPos/1 -> Engine Control Module (ECM)/15(IntkSwirlVlvPos)
  WgAreaPct/1 -> Engine Control Module (ECM)/6(WgAreaPct)
  ThrPosPct/1 -> Engine Control Module (ECM)/5(ThrPosPct)
  EgrVlvAreaPct/1 -> Engine Control Module (ECM)/10(EgrVlvAreaPct)
  TurboRackPos/1 -> Engine Control Module (ECM)/9(TurboRackPos)
  Mat/1 -> Engine Control Module (ECM)/4(Mat)
  Map/1 -> Engine Control Module (ECM)/3(Map)
  EngSpd/1 -> Engine Control Module (ECM)/2(EngSpd)
  TrqCmd/1 -> Engine Control Module (ECM)/1(TrqCmd)
  AmbPrs/1 -> Engine Control Module (ECM)/17(AmbPrs)
  TurboSpd/1 -> Engine Control Module (ECM)/16(TurboSpd)
  ExhCamPhase/1 -> Engine Control Module (ECM)/8(ExhCamPhase)
  IntkCamPhase/1 -> Engine Control Module (ECM)/7(IntkCamPhase)
  IgSw/1 -> Engine Control Module (ECM)/18(IgSw)
  Ect/1 -> Engine Control Module (ECM)/20(Ect)
  Engine Control Module (ECM)/1(ThrPosPctCmd) -> ThrPosPctCmd/1
  Engine Control Module (ECM)/2(WgAreaPctCmd) -> WgAreaPctCmd/1
  Engine Control Module (ECM)/3(InjPw) -> InjPw/1
  Engine Control Module (ECM)/4(FuelMainSoi) -> FuelMainSoi/1
  Engine Control Module (ECM)/5(SpkAdv) -> SpdAdv/1
  Engine Control Module (ECM)/6(IntkCamPhaseCmd) -> IntkCamPhaseCmd/1
  Engine Control Module (ECM)/7(ExhCamPhaseCmd) -> ExhCamPhaseCmd/1
  Engine Control Module (ECM)/8(TurboRackPosCmd) -> TurboRackPosCmd/1
  Engine Control Module (ECM)/9(EgrVlvAreaPctCmd) -> EgrVlvAreaPctCmd/1
  Engine Control Module (ECM)/10(VarCompRatioPosCmd) -> VarCompRatioPosCmd/1
  Engine Control Module (ECM)/11(IntkVlvLiftCmd) -> IntkVlvLiftCmd/1
  Engine Control Module (ECM)/12(VarIntkRunLenCmd) -> VarIntkRunLenCmd/1
  Engine Control Module (ECM)/13(ClsdLpFuelMult) -> ClsdLpFuelMult/1
  Engine Control Module (ECM)/14(IntkSwirlVlvPosCmd) -> IntkSwirlVlvPosCmd/1
  Engine Control Module (ECM)/15(TrqCmdISC) -> TrqCmdISC/1
  Engine Control Module (ECM)/16(LoadCmd) -> LoadCmd/1
  Engine Control Module (ECM)/17(EstIntkPortFlw) -> EstIntkPortFlw/1
  EgrVlvDeltaPrs/1 -> Engine Control Module (ECM)/21(EgrVlvDeltaPrs)
  EgrVlvInTemp/1 -> Engine Control Module (ECM)/22(EgrVlvInTemp)
  Iat/1 -> Engine Control Module (ECM)/19(Iat)

== system HevMmReferenceApplication/Longitudinal Driver/Longitudinal Driver ==
  Vref : Inport
  Vfdbk : Inport  Port=2
  Bus Creator1 : BusCreator  Inputs=2
  Bus Selector : BusSelector  OutputSignals=Veh.xdot
  Constant : Constant  Value=false
  Data Type Conversion : DataTypeConversion  OutDataTypeStr=boolean
  Ground : Ground
  Ignition Switch Profile : Subsystem  Tag=STV Subsys  LoadFcn=sigbuilder_block('load');  StartFcn=sigbuilder_block('start');  StopFcn=sigbuilder_block('stop');  ClipboardFcn=sigbuilder_block('clipboard');  mask(Sigbuilder block){tuvar=[0:10]}
      mask help: Simulink:masks:SigbuilderBlock_MD
      mask init:
      | if ~strcmp(get_param(bdroot(gcbh),'SimulationStatus'),'stopped') tuvar = sigbuilder_block('maskInit'); end
      settings: CopyFcn=sigbuilder_block('copy');  DeleteFcn=sigbuilder_block('delete');  ModelCloseFcn=sigbuilder_block('modelClose');  PreSaveFcn=sigbuilder_block('preSave');  PauseFcn=sigbuilder_block('pause');  ContinueFcn=sigbuilder_block('continue');  NameChangeFcn=sigbuilder_block('namechange');  OpenFcn=sigbuilder_block('open',[595.8 176.4 550.8 322.2 ]);  CloseFcn=sigbuilder_block('close');
      mask Display: plot(0, 0, 100, 100,[2, 2, 32, 32, 2], [68, 8, 8, 68, 68],[32, 2], [38, 38], [32, 19, 2],[53, 60, 44], [32, 17, 17, 2],[16, 16, 31, 31]);txt = getActiveGroup(gcbh);text(2, 100, txt,'verticalAlignment', 'top');
  Longitudinal Driver Model : autolibshared/Longitudinal Driver  extAccelOvr=off  extDecelOvr=off  extAccelHld=off  extDecelHld=off  extAccelZero=off  extDecelZero=off  cntrlType=Predictive  shftType=Reverse, Neutral, Drive  velUnits=m/s  gearOut=off  Kp=1  Ki=1  Kff=.1  Kg=0  VehVelVec=[0 100]  KffVec=[.1 .1]  KpVec=[10 10]  KiVec=[5 5]  KgVec=[0 0]  m=1500  Kpt=10000  tau=0.12  L=4  aR=160  bR=1  cR=0.36  g=9.81  vnom=5  Kaw=1  tauerr=0.01  tauPt=2  GearInit=0  tShift=.1  pdlVec=[0.1 0.4 0.5 0.9]  upShftTbl=[-1 12.9375 26.4375 39.9375 51.18749999999999 62.4375 72.84375 83.25;-1 16.3125 29.8125 43.3125 54.5624 65.8125 76.78125 87.75;-1 19.6875 33.1875 46.68749999999999 57.9375 69.1875 80.71875 92.25;-1 33 52.5 77.25 100.5 138.75 161.875 185]  dwnShftTbl=[1 9.5625 23.0625 36.5625 47.8125 59.0625 68.90625 78.75;1 12.9375 26.4375 39.9375 51.18749999999999 62.4375 72.84375 83.25;1 16.3125 29.8125 43.3125 54.562499 65.8125 76.78125 87.75;1 19.6875 33.1875 46.68749999999999 57.9375 69.1875 80.71875 92.25]  tClutch=.5  tRev=.5  tPark=120  aMode=1  UpGearVec="[0  1  2  3  4  5  6  7]"  DownGearVec="[1  2  3  4  5  6  7  8]"
      settings: SourceProductBaseCode=PW,MT,VE,VP
  Manual Switch : ManualSwitch
  Terminator : Terminator
  Terminator1 : Terminator
  OpCmds : Outport  VectorParamsAs1DForOutWhenUnconnected=off
  wires:
  Vfdbk/1 -> Bus Selector/1
  Ground/1 -> Longitudinal Driver Model/3
  Bus Selector/1 -> Longitudinal Driver Model/2  "<xdot>"
  Bus Creator1/1 -> OpCmds/1
  Longitudinal Driver Model/1 -> Bus Creator1/1  "Info"
  Longitudinal Driver Model/2 -> Terminator/1  "Acc"
  Ignition Switch Profile/1(IGSW) -> Data Type Conversion/1
  Data Type Conversion/1 -> Manual Switch/2
  Manual Switch/1 -> Bus Creator1/2  "IgSw"
  Vref/1 -> Longitudinal Driver Model/1  "xdotref"
  Longitudinal Driver Model/3 -> Terminator1/1  "Dec"
  Constant/1 -> Manual Switch/1

== system HevMmReferenceApplication/Longitudinal Driver/Open Loop ==
  note: This subsystem is provided to disable the driver subsystem and expose the driver interface.
      |
      | The interface can:
      | - be connected with dashboard UI blocks or 3rd party hardware
      | - provide application specific pre-programmed event or time based signals
      | - be driven by recorded operator signals for tuning, troubleshooting and model validation
  Bus Creator1 : BusCreator  Inputs=2
  Bus Creator2 : BusCreator  Inputs=8
  Constant : Constant  Value=false
  Constant{1..4} (4 alike) : Constant  Value=0
  Data Type Conversion : DataTypeConversion  OutDataTypeStr=boolean
  Ground{,1..3} (4 alike) : Ground
  Ignition Switch Profile : Subsystem  Tag=STV Subsys  LoadFcn=sigbuilder_block('load');  StartFcn=sigbuilder_block('start');  StopFcn=sigbuilder_block('stop');  ClipboardFcn=sigbuilder_block('clipboard');  mask(Sigbuilder block){tuvar=[0:10]}
      mask help: Simulink:masks:SigbuilderBlock_MD
      mask init:
      | if ~strcmp(get_param(bdroot(gcbh),'SimulationStatus'),'stopped') tuvar = sigbuilder_block('maskInit'); end
      settings: CopyFcn=sigbuilder_block('copy');  DeleteFcn=sigbuilder_block('delete');  ModelCloseFcn=sigbuilder_block('modelClose');  PreSaveFcn=sigbuilder_block('preSave');  PauseFcn=sigbuilder_block('pause');  ContinueFcn=sigbuilder_block('continue');  NameChangeFcn=sigbuilder_block('namechange');  OpenFcn=sigbuilder_block('open',[595.8 176.4 550.8 322.2 ]);  CloseFcn=sigbuilder_block('close');
      mask Display: plot(0, 0, 100, 100,[2, 2, 32, 32, 2], [68, 8, 8, 68, 68],[32, 2], [38, 38], [32, 19, 2],[53, 60, 44], [32, 17, 17, 2],[16, 16, 31, 31]);txt = getActiveGroup(gcbh);text(2, 100, txt,'verticalAlignment', 'top');
  Manual Switch : ManualSwitch
  OpCmds : Outport  VectorParamsAs1DForOutWhenUnconnected=off
  wires:
  Constant4/1 -> Bus Creator2/4  "Clutch"
  Ground/1 -> Bus Creator2/5  "Err"
  Constant2/1 -> Bus Creator2/2  "Decel"
  Constant3/1 -> Bus Creator2/3  "Gear"
  Constant1/1 -> Bus Creator2/1  "Accel"
  Ground2/1 -> Bus Creator2/7  "ErrMax"
  Bus Creator2/1 -> Bus Creator1/1  "Info"
  Ground1/1 -> Bus Creator2/6  "ErrSqrSum"
  Ground3/1 -> Bus Creator2/8  "ErrMin"
  Ignition Switch Profile/1(IGSW) -> Data Type Conversion/1
  Manual Switch/1 -> Bus Creator1/2  "IgSw"
  Bus Creator1/1 -> OpCmds/1
  Constant/1 -> Manual Switch/1
  Data Type Conversion/1 -> Manual Switch/2

== system HevMmReferenceApplication/Passenger Car/Drivetrain Output ==
  VehSpd : Inport
  "EngSpd " : Inport  Port=2
  EngCltchState : Inport  Port=3
  GenSpd : Inport  Port=4
  MotSpd : Inport  Port=5
  EngCltchOutSpd : Inport  Port=6
  Bus Creator1 : BusCreator  Inputs=5
  Bus Creator3 : BusCreator  Inputs=1
  VehFdbk : Outport  VectorParamsAs1DForOutWhenUnconnected=off
  EngFdbk : Outport  Port=2  VectorParamsAs1DForOutWhenUnconnected=off
  wires:
  Bus Creator1/1 -> VehFdbk/1  "VehFdbk"
  VehSpd/1 -> Bus Creator1/1
  "EngSpd "/1 -> Bus Creator3/1  "EngSpd"
  Bus Creator3/1 -> EngFdbk/1  "EngFdbk"
  EngCltchState/1 -> Bus Creator1/2  "EngCltchState"
  GenSpd/1 -> Bus Creator1/3  "GenSpd"
  MotSpd/1 -> Bus Creator1/4  "MotSpd"
  EngCltchOutSpd/1 -> Bus Creator1/5  "EngCltchOutSpd"

== system HevMmReferenceApplication/Passenger Car/Drivetrain Plant Input ==
  Ctrl : Inport
  EngFdbk : Inport  Port=2
  ElecFdbk : Inport  Port=3
  Env : Inport  Port=4
  Bus Selector : BusSelector  OutputSignals=PtCtrl.EngCltchCmd,PtCtrl.BrakeCmd
  Bus Selector1 : BusSelector  OutputSignals=GenTrq,MotTrq
  Bus Selector2 : BusSelector  OutputSignals=EngTrq
  Bus Selector3 : BusSelector  OutputSignals=Ground.Grade,Wind.wind_x
  Engine Flex Plate Dynamics : TransferFcn  Denominator=[0.05 1]
  Rate Transition3 : RateTransition  Deterministic=off
  Rate Transition4 : RateTransition  Deterministic=off
  EngCltchCmd : Outport  VectorParamsAs1DForOutWhenUnconnected=off
  EngineTrq : Outport  Port=2  VectorParamsAs1DForOutWhenUnconnected=off
  GenTrq : Outport  Port=3  VectorParamsAs1DForOutWhenUnconnected=off
  MotTrq : Outport  Port=4  VectorParamsAs1DForOutWhenUnconnected=off
  Grade Angle : Outport  Port=5  VectorParamsAs1DForOutWhenUnconnected=off
  Wind Vel : Outport  Port=6  VectorParamsAs1DForOutWhenUnconnected=off
  BrakeCmd : Outport  Port=7  VectorParamsAs1DForOutWhenUnconnected=off
  wires:
  Ctrl/1 -> Bus Selector/1
  Bus Selector2/1 -> Engine Flex Plate Dynamics/1  "<EngTrq>"
  EngFdbk/1 -> Bus Selector2/1
  Bus Selector/2 -> Rate Transition3/1  "<BrakeCmd>"
  Bus Selector/1 -> Rate Transition4/1  "<EngCltchCmd>"
  Rate Transition4/1 -> EngCltchCmd/1  "EngCltchCmd"
  Rate Transition3/1 -> BrakeCmd/1  "BrakeCntrlCmd"
  ElecFdbk/1 -> Bus Selector1/1
  Engine Flex Plate Dynamics/1 -> EngineTrq/1
  Env/1 -> Bus Selector3/1
  Bus Selector1/1 -> GenTrq/1  "<GenTrq>"
  Bus Selector1/2 -> MotTrq/1  "<MotTrq>"
  Bus Selector3/1 -> Grade Angle/1  "<Grade>"
  Bus Selector3/2 -> Wind Vel/1  "<wind_x>"

== system HevMmReferenceApplication/Passenger Car/Electric Plant ==
  GenTrqCmd : Inport
  MotTrqCmd : Inport  Port=2
  GenSpd : Inport  Port=3
  MotSpd : Inport  Port=4
  AmbTemp : Inport  Port=5
  Battery : ModelReference  ModelNameDialog=BattHevMm.slx  SimulationMode=Normal  ModelReferenceVersion=1.357
  Battery Discharge Dynamics : TransferFcn  Denominator=[0.05 1]
  Bus Current : Sum
  Generator : Subsystem  Variant=on  VariantControlMode=Label  LabelModeActiveChoice=GenMapped
  Generator Coupling Dynamics : TransferFcn  Denominator=[0.05 1]
  Motor : Subsystem  Variant=on  VariantControlMode=Label  LabelModeActiveChoice=MotMapped
  Motor Coupling Dynamics : TransferFcn  Denominator=[0.05 1]
  Product : Product
  Product1 : Product
  Product2 : Product
  BattSoc : Outport  VectorParamsAs1DForOutWhenUnconnected=off
  BattPwr : Outport  Port=2  VectorParamsAs1DForOutWhenUnconnected=off
  BattCrnt : Outport  Port=3  VectorParamsAs1DForOutWhenUnconnected=off
  GenPwrElec : Outport  Port=4  VectorParamsAs1DForOutWhenUnconnected=off
  GenPwrMech : Outport  Port=5  VectorParamsAs1DForOutWhenUnconnected=off
  GenTrq : Outport  Port=6  VectorParamsAs1DForOutWhenUnconnected=off
  MotTrq : Outport  Port=7  VectorParamsAs1DForOutWhenUnconnected=off
  wires:
  Product/1 -> GenPwrMech/1  "GenPwrMech"
  Bus Current/1 -> Battery Discharge Dynamics/1, BattCrnt/1  "BattCrnt"
  Battery/2 -> Generator/3(BusVolt), Product1/2, Motor/3(BusVolt), Product2/1
  Product1/1 -> GenPwrElec/1  "GenPwrElec"
  Battery/1 -> BattSoc/1  "BattSoc"
  MotSpd/1 -> Motor/2(MotSpd)
  Generator/2(GenCurnt) -> Product1/1, Bus Current/1
  MotTrqCmd/1 -> Motor/1(MotTrqCmd)
  GenTrqCmd/1 -> Generator/1(GenTrqCmd)
  AmbTemp/1 -> Battery/2
  Product2/1 -> BattPwr/1  "BattPwr"
  GenSpd/1 -> Generator/2(GenSpd), Product/1
  Motor/1(MotTrq) -> Motor Coupling Dynamics/1
  Generator/1(GenTrq) -> Generator Coupling Dynamics/1
  Generator Coupling Dynamics/1 -> Product/2, GenTrq/1  "GenTrq"
  Motor/2(MotCurnt) -> Bus Current/2
  Battery Discharge Dynamics/1 -> Product2/2, Battery/1
  Motor Coupling Dynamics/1 -> MotTrq/1  "MotTrq"

== system HevMmReferenceApplication/Passenger Car/Electric Plant Input ==
  Ctrl : Inport
  Veh : Inport  Port=2
  Env : Inport  Port=3
  Bus Selector : BusSelector  OutputSignals=PtCtrl.GenTrqCmd,PtCtrl.MotTrqCmd
  Bus Selector1 : BusSelector  OutputSignals=GenSpd,MotSpd
  Bus Selector2 : BusSelector  OutputSignals=Temp
  Rate Transition4 : RateTransition  Deterministic=off
  Rate Transition5 : RateTransition  Deterministic=off
  GenTrqCmd : Outport  VectorParamsAs1DForOutWhenUnconnected=off
  MotTrqCmd : Outport  Port=2  VectorParamsAs1DForOutWhenUnconnected=off
  GenSpd : Outport  Port=3  VectorParamsAs1DForOutWhenUnconnected=off
  MotSpd : Outport  Port=4  VectorParamsAs1DForOutWhenUnconnected=off
  AmbTemp : Outport  Port=5  VectorParamsAs1DForOutWhenUnconnected=off
  wires:
  Rate Transition5/1 -> MotTrqCmd/1  "MotTrqCmd"
  Rate Transition4/1 -> GenTrqCmd/1  "GenTrqCmd"
  Ctrl/1 -> Bus Selector/1
  Bus Selector/2 -> Rate Transition5/1  "<MotTrqCmd>"
  Bus Selector/1 -> Rate Transition4/1  "<GenTrqCmd>"
  Veh/1 -> Bus Selector1/1
  Env/1 -> Bus Selector2/1
  Bus Selector1/1 -> GenSpd/1  "<GenSpd>"
  Bus Selector1/2 -> MotSpd/1  "<MotSpd>"
  Bus Selector2/1 -> AmbTemp/1  "<Temp>"

== system HevMmReferenceApplication/Passenger Car/Electric Plant Output ==
  BattSoc : Inport
  BattPwr : Inport  Port=2
  BattCrnt : Inport  Port=3
  GenPwrElec : Inport  Port=4
  GenPwrMech : Inport  Port=5
  GenTrq : Inport  Port=6
  MotTrq : Inport  Port=7
  Bus Creator1 : BusCreator  Inputs=7
  ElecFdbk : Outport  VectorParamsAs1DForOutWhenUnconnected=off
  wires:
  Bus Creator1/1 -> ElecFdbk/1  "ElecFdbk"
  BattPwr/1 -> Bus Creator1/2
  BattSoc/1 -> Bus Creator1/1
  BattCrnt/1 -> Bus Creator1/3
  GenTrq/1 -> Bus Creator1/6
  MotTrq/1 -> Bus Creator1/7
  GenPwrElec/1 -> Bus Creator1/4
  GenPwrMech/1 -> Bus Creator1/5
